simulink model "ModeloMelhor"  (R2021a)
settings: Solver=ode4  StartTime=0.0  StopTime=10.0  FixedStep=0.005  RelTol=1e-3  EnableMultiTasking=on
undefined symbols (not defined in the file): Angle, Axis
libraries: robotcorelib x5, simulink_extras x2, aerolibutil x1, sharedutil x1, sharedtransform x1, vrlib x1
settings Model: Creator=Usuario  LastModifiedBy=Usuario
settings OptimizationCC: EnhancedBackFolding=on  PassReuseOutputArgsAs=Individual arguments  ZeroExternalMemoryAtStartup=off  ZeroInternalMemoryAtStartup=off  MaxStackSize=64  OptimizeBlockOrder=speed  DifferentSizesBufferReuse=on  OptimizationCustomize=off  EfficientTunableParamExpr=on
settings DebuggingCC: ParameterTunabilityLossMsg=error
settings HardwareCC: ProdBitPerPointer=32  ProdBitPerSizeT=32  ProdBitPerPtrDiffT=32  ProdLargestAtomicInteger=Long  ProdLargestAtomicFloat=Double  ProdWordSize=32  ProdHWDeviceType=ARM Compatible->ARM Cortex
settings SFSimCC: MATLABDynamicMemAlloc=off
settings RTWCC: SystemTargetFile=ert.tlc  HardwareBoard=STM32F4-Discovery  TemplateMakefile=ert_default_tmf  Toolchain=GNU Tools for ARM Embedded Processors
settings CodeAppCC: ForceParamTrailComments=on  IgnoreCustomStorageClasses=off  OperatorAnnotations=on  SimulinkDataObjDesc=on  SFDataObjDesc=on  InsertBlockDesc=on
settings ERTTargetCC: CodeReplacementLibrary=ARM Cortex-M (Optimized)  ExtModeTransport=1  ExtModeMexFile=ext_serial_win32_comm

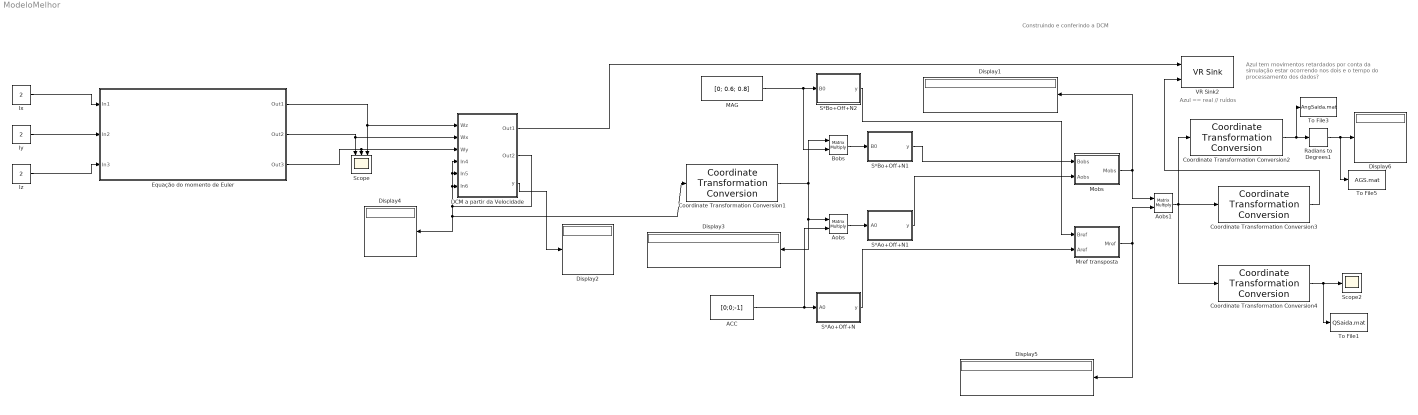
== system ModeloMelhor ==
  note: Azul == real // ruídos
  note: Construindo e conferindo a DCM
  note: Azul tem movimentos retardados por conta da
      | simulação estar ocorrendo nos dois e o tempo do
      | processamento dos dados?
  ACC : Constant  Value=[0;0;-1]
  Aobs : Product  Multiplication=Matrix(*)
  Aobs1 : Product  Multiplication=Matrix(*)
  Bobs : Product  Multiplication=Matrix(*)
  Coordinate Transformation Conversion1 : robotcorelib/Coordinate Transformation Conversion  InputRepresentation=Quaternion  InputEulerSequence=ZYX  ShowTrVecInputPort=on  OutputRepresentation=Rotation Matrix  OutputEulerSequence=ZYX  ShowTrVecOutputPort=on  SimulateUsing=Interpreted execution
      settings: SourceProductBaseCode=NV,RO,RR,UV
  Coordinate Transformation Conversion2 : robotcorelib/Coordinate Transformation Conversion  InputRepresentation=Rotation Matrix  InputEulerSequence=ZYX  ShowTrVecInputPort=on  OutputRepresentation=Euler Angles  OutputEulerSequence=ZYX  ShowTrVecOutputPort=on  SimulateUsing=Interpreted execution
      settings: SourceProductBaseCode=NV,RO,RR,UV
  Coordinate Transformation Conversion3 : robotcorelib/Coordinate Transformation Conversion  InputRepresentation=Rotation Matrix  InputEulerSequence=ZYX  ShowTrVecInputPort=on  OutputRepresentation=Axis-Angle  OutputEulerSequence=ZYX  ShowTrVecOutputPort=on  SimulateUsing=Interpreted execution
      settings: SourceProductBaseCode=NV,RO,RR,UV
  Coordinate Transformation Conversion4 : robotcorelib/Coordinate Transformation Conversion  InputRepresentation=Rotation Matrix  InputEulerSequence=ZYX  ShowTrVecInputPort=on  OutputRepresentation=Quaternion  OutputEulerSequence=ZYX  ShowTrVecOutputPort=on  SimulateUsing=Interpreted execution
      settings: SourceProductBaseCode=NV,RO,RR,UV
  DCM a partir da Velocidade : Subsystem
  Display{1..6} (6 alike) : Display
  Equação do momento de Euler : Subsystem
  Ix : Constant  Value=2
  Iy : Constant  Value=2
  Iz : Constant  Value=2
  MAG : Constant  Value=[0; 0.6; 0.8]
  Mobs : MATLAB Function  TreatAsAtomicUnit=on
  Mref transposta : MATLAB Function  TreatAsAtomicUnit=on
  Radians to Degrees1 : simulink_extras/Transformations/Radians to Degrees
  S*Ao+Off+N : MATLAB Function  TreatAsAtomicUnit=on
  S*Ao+Off+N1 : MATLAB Function  TreatAsAtomicUnit=on
  S*Bo+Off+N1 : MATLAB Function  TreatAsAtomicUnit=on
  S*Bo+Off+N2 : MATLAB Function  TreatAsAtomicUnit=on
  Scope : Scope  NumInputPorts=3
  Scope2 : Scope
  To File1 : ToFile  Filename=QSaida.mat  MatrixName=Que
  To File3 : ToFile  Filename=AngSaida.mat  MatrixName=AngS
  To File5 : ToFile  Filename=AGS.mat  MatrixName=AGS
  VR Sink2 : vrlib/VR Sink  InstantiateOnLoad=on  SampleTime=-1  ViewEnable=on  RemoteChange=off  RemoteView=off  FieldsWritten=Modelo.rotation.4.1.1.double#Real.rotation.4.1.1.double  WorldFileName=2 cubos.x3d  AutoView=off  VideoDimensions=[]  AllowVariableSize=off
  wires:
  Coordinate Transformation Conversion1/1 -> Aobs/1, Display3/1, Bobs/1
  MAG/1 -> Bobs/2, S*Bo+Off+N2/1(B0)
  ACC/1 -> Aobs/2, S*Ao+Off+N/1(A0)
  Bobs/1 -> S*Bo+Off+N1/1(B0)
  Aobs/1 -> S*Ao+Off+N1/1(A0)
  S*Ao+Off+N/1(y) -> Mref transposta/2(Aref)
  Mobs/1(Mobs) -> Aobs1/1, Display1/1
  Mref transposta/1(Mref) -> Aobs1/2, Display5/1
  S*Bo+Off+N2/1(y) -> Mref transposta/1(Bref)
  S*Bo+Off+N1/1(y) -> Mobs/1(Bobs)
  S*Ao+Off+N1/1(y) -> Mobs/2(Aobs)
  Aobs1/1 -> Coordinate Transformation Conversion4/1, Coordinate Transformation Conversion3/1, Coordinate Transformation Conversion2/1
  Radians to Degrees1/1 -> To File5/1, Display6/1
  Coordinate Transformation Conversion2/1 -> To File3/1, Radians to Degrees1/1
  Coordinate Transformation Conversion3/1 -> VR Sink2/2
  Coordinate Transformation Conversion4/1 -> To File1/1, Scope2/1
  Equação do momento de Euler/2(Out2) -> Scope/1, DCM a partir da Velocidade/2(Wx)
  Equação do momento de Euler/1(Out1) -> Scope/3, DCM a partir da Velocidade/1(Wz)
  Equação do momento de Euler/3(Out3) -> Scope/2, DCM a partir da Velocidade/3(Wy)
  Ix/1 -> Equação do momento de Euler/1(In1)
  Iy/1 -> Equação do momento de Euler/2(In2)
  Iz/1 -> Equação do momento de Euler/3(In3)
  DCM a partir da Velocidade/2(Out2) -> Coordinate Transformation Conversion1/1, Display4/1, DCM a partir da Velocidade/5(In5), DCM a partir da Velocidade/4(In4), DCM a partir da Velocidade/6(In6)
  DCM a partir da Velocidade/1(Out1) -> VR Sink2/1
  DCM a partir da Velocidade/3(y) -> Display2/1

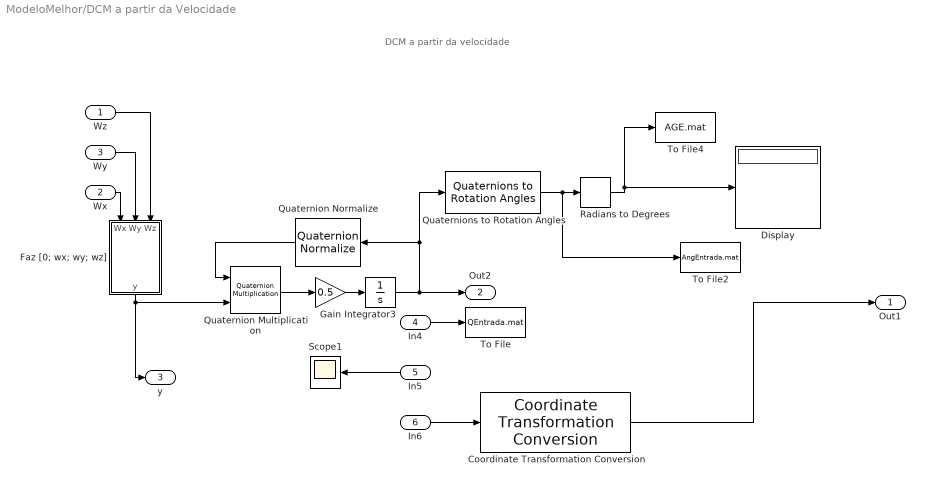
== system ModeloMelhor/DCM a partir da Velocidade ==
  note: DCM a partir da velocidade
  Wz : Inport
  Wx : Inport  Port=2
  Wy : Inport  Port=3
  In4 : Inport  Port=4
  In5 : Inport  Port=5
  In6 : Inport  Port=6
  Coordinate Transformation Conversion : robotcorelib/Coordinate Transformation Conversion  InputRepresentation=Quaternion  InputEulerSequence=ZYX  ShowTrVecInputPort=on  OutputRepresentation=Axis-Angle  OutputEulerSequence=ZYX  ShowTrVecOutputPort=on  SimulateUsing=Interpreted execution
      settings: SourceProductBaseCode=NV,RO,RR,UV
  Display : Display
  Faz [0; wx; wy; wz] : MATLAB Function  TreatAsAtomicUnit=on
  Gain : Gain  Gain=0.5
  Integrator3 : Integrator  InitialCondition=[0 0 0 1]
  Quaternion Multiplication : aerolibutil/Quaternion Multiplication
  Quaternion Normalize : sharedutil/Quaternion Normalize  aMode=aMode
      settings: SourceProductBaseCode=AE,PW,DR,MT,UV,VE
  Quaternions to Rotation Angles : sharedtransform/Quaternions to Rotation Angles  rotationOrder=ZYX  aMode=aMode
      settings: SourceProductBaseCode=AE,PW,DR,MT,UV,VE
  Radians to Degrees : simulink_extras/Transformations/Radians to Degrees
  Scope1 : Scope
  To File : ToFile  Filename=QEntrada.mat  MatrixName=qu
  To File2 : ToFile  Filename=AngEntrada.mat  MatrixName=AngE
  To File4 : ToFile  Filename=AGE.mat  MatrixName=AGE
  Out1 : Outport
  Out2 : Outport  Port=2
  y : Outport  Port=3
  wires:
  Integrator3/1 -> Out2/1, Quaternions to Rotation Angles/1, Quaternion Normalize/1
  Faz [0; wx; wy; wz]/1(y) -> y/1, Quaternion Multiplication/2
  Gain/1 -> Integrator3/1
  Quaternions to Rotation Angles/1 -> To File2/1, Radians to Degrees/1
  Quaternion Multiplication/1 -> Gain/1
  Radians to Degrees/1 -> To File4/1, Display/1
  In4/1 -> To File/1
  Quaternion Normalize/1 -> Quaternion Multiplication/1
  In6/1 -> Coordinate Transformation Conversion/1
  Wy/1 -> Faz [0; wx; wy; wz]/2(Wy)
  Wz/1 -> Faz [0; wx; wy; wz]/3(Wz)
  In5/1 -> Scope1/1
  Coordinate Transformation Conversion/1 -> Out1/1
  Wx/1 -> Faz [0; wx; wy; wz]/1(Wx)

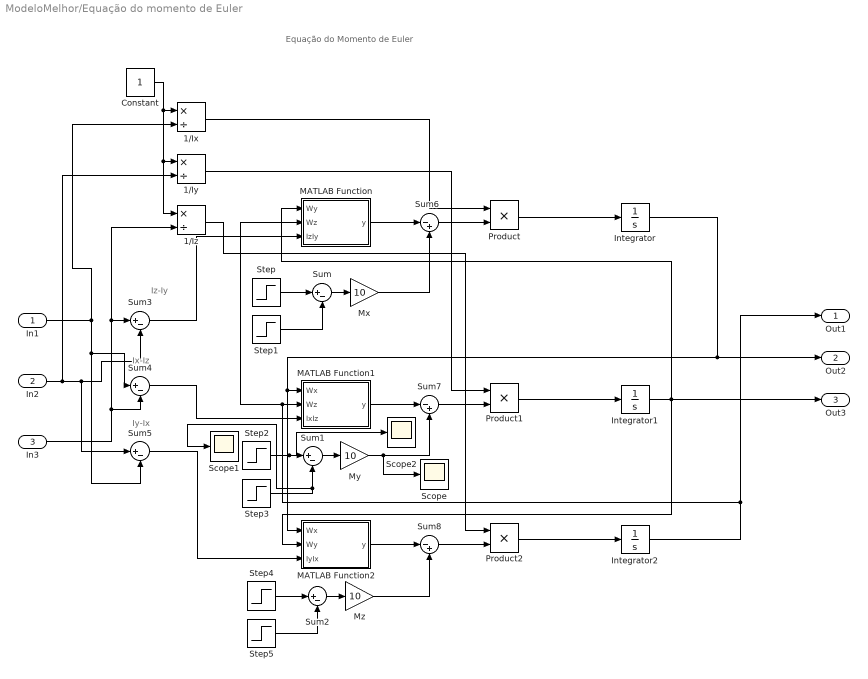
== system ModeloMelhor/Equação do momento de Euler ==
  note: Equação do Momento de Euler
  note: Ix-Iz
  note: Iz-Iy
  note: Iy-Ix
  In1 : Inport
  In2 : Inport  Port=2
  In3 : Inport  Port=3
  1/Ix : Product  Inputs=*/
  1/Iy : Product  Inputs=*/
  1/Iz : Product  Inputs=*/
  Constant : Constant
  Integrator : Integrator
  Integrator1 : Integrator
  Integrator2 : Integrator
  MATLAB Function : MATLAB Function  TreatAsAtomicUnit=on
  MATLAB Function1 : MATLAB Function  TreatAsAtomicUnit=on
  MATLAB Function2 : MATLAB Function  TreatAsAtomicUnit=on
  Mx : Gain  Gain=10
  My : Gain  Gain=10
  Mz : Gain  Gain=10
  Product : Product
  Product1 : Product
  Product2 : Product
  Scope : Scope
  Scope1 : Scope
  Scope2 : Scope
  Step : Step  SampleTime=0
  Step1 : Step  Time=1.1  SampleTime=0
  Step2 : Step  Time=2  SampleTime=0
  Step3 : Step  Time=2.1  SampleTime=0
  Step4 : Step  Time=3  SampleTime=0
  Step5 : Step  Time=3.1  SampleTime=0
  Sum{,1..5} (6 alike) : Sum  Inputs=|+-
  Sum6 : Sum  Inputs=|-+
  Sum7 : Sum  Inputs=|-+
  Sum8 : Sum  Inputs=|-+
  Out1 : Outport
  Out2 : Outport  Port=2
  Out3 : Outport  Port=3
  wires:
  Constant/1 -> 1/Iz/1, 1/Iy/1, 1/Ix/1
  Mz/1 -> Sum8/2
  My/1 -> Scope/1, Sum7/2
  In3/1 -> Sum4/2, 1/Iz/2, Sum3/1
  Mx/1 -> Sum6/2
  In2/1 -> Sum3/2, Sum5/1, 1/Iy/2
  Sum4/1 -> MATLAB Function1/3(IxIz)
  Sum3/1 -> MATLAB Function/3(IzIy)
  1/Ix/1 -> Product/1
  1/Iz/1 -> Product2/1
  Sum8/1 -> Product2/2
  Integrator1/1 -> MATLAB Function/1(Wy), Out3/1, MATLAB Function2/2(Wy)
  Step4/1 -> Sum2/1
  Integrator2/1 -> Out1/1, MATLAB Function/2(Wz), MATLAB Function1/2(Wz)
  Sum/1 -> Mx/1
  Product1/1 -> Integrator1/1
  In1/1 -> Sum5/2, Sum4/1, 1/Ix/2
  MATLAB Function2/1(y) -> Sum8/1
  Step2/1 -> Scope2/1, Sum1/1
  Sum1/1 -> My/1
  Step1/1 -> Sum/2
  Integrator/1 -> MATLAB Function2/1(Wx), MATLAB Function1/1(Wx), Out2/1
  Sum2/1 -> Mz/1
  1/Iy/1 -> Product1/1
  Product/1 -> Integrator/1
  Sum7/1 -> Product1/2
  MATLAB Function/1(y) -> Sum6/1
  Sum5/1 -> MATLAB Function2/3(IyIx)
  Step5/1 -> Sum2/2
  MATLAB Function1/1(y) -> Sum7/1
  Product2/1 -> Integrator2/1
  Step3/1 -> Scope1/1, Sum1/2
  Step/1 -> Sum/1
  Sum6/1 -> Product/2

== matlab function ModeloMelhor/Equação do momento de Euler/MATLAB Function ==
  data: Wy input; y output; Wz input; IzIy input
function y = fcn(Wy, Wz, IzIy)

y = Wy*Wz*IzIy;

== matlab function ModeloMelhor/Equação do momento de Euler/MATLAB Function2 ==
  data: Wx input; Wy input; y output; IyIx input
function y = fcn(Wx, Wy, IyIx)

y = Wx*Wy*IyIx;

== matlab function ModeloMelhor/DCM a partir da Velocidade/Faz [0; wx; wy; wz] ==
  data: Wx input; y output; Wy input; Wz input
function y = fcn(Wx,Wy,Wz)

y = [0;Wx;Wy;Wz];

== matlab function ModeloMelhor/S*Ao+Off+N ==
  data: A0 input; y output
function y = fcn(A0)
Vs = ones(3,1);
S = diag(Vs);
Off = 0; 
N = 0; %rand(3,1);
Aref = S*A0+Off+N;
y = Aref;

== matlab function ModeloMelhor/S*Bo+Off+N1 ==
  data: B0 input; y output
function y = fcn(B0)
Vs = ones(3,1);
S = diag(Vs);
Off = 0; 
N = 0; %rand(3,1);
Bref = S*B0+Off+N;
y = Bref;

== matlab function ModeloMelhor/S*Ao+Off+N1 ==
  data: A0 input; y output
function y = fcn(A0)
Vs = ones(3,1);
S = diag(Vs);
Off = 0; 
N = 0; %rand(3,1);
Aref = S*A0+Off+N;
y = Aref;

== matlab function ModeloMelhor/S*Bo+Off+N2 ==
  data: B0 input; y output
function y = fcn(B0)
S = diag([1.01 0.99 0.98]);
Off = [-0.01 0.025 0.09]'; 
N = 0; %rand(3,1);
Bref = S*B0+Off+N;
y = Bref;

== matlab function ModeloMelhor/Mobs ==
  data: Bobs input; Mobs output; Aobs input
function Mobs = fcn(Bobs, Aobs)

r1=Bobs/norm(Bobs);
r2=cross(r1,Aobs);
r2=r2/norm(r2);
r3=cross(r1,r2);
r3=r3/norm(r3);

Mobs=[r1, r2, r3];

== matlab function ModeloMelhor/Mref transposta ==
  data: Bref input; Mref output; Aref input
function Mref = fcn(Bref, Aref)

r1=Bref/norm(Bref);
r2=cross(r1,Aref);
r2=r2/norm(r2);
r3=cross(r1,r2);
r3=r3/norm(r3);

Mref=[r1, r2, r3]';

== matlab function ModeloMelhor/Equação do momento de Euler/MATLAB Function1 ==
  data: Wx input; y output; Wz input; IxIz input
function y = fcn(Wx, Wz, IxIz)

y = Wx*Wz*IxIz;
